simulink model "ned2lla_block"  (R2024b)
settings: Solver=VariableStepAuto  StartTime=0.0  StopTime=15  RelTol=1e-3
libraries: simulink x6, aerolibfltsims x1
settings Model: Creator=victo  LastModifiedBy=victo

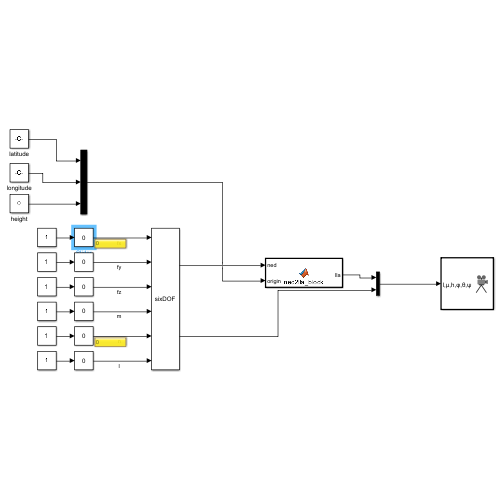
[thumbnail: Simulink's stored preview of the top-level diagram]
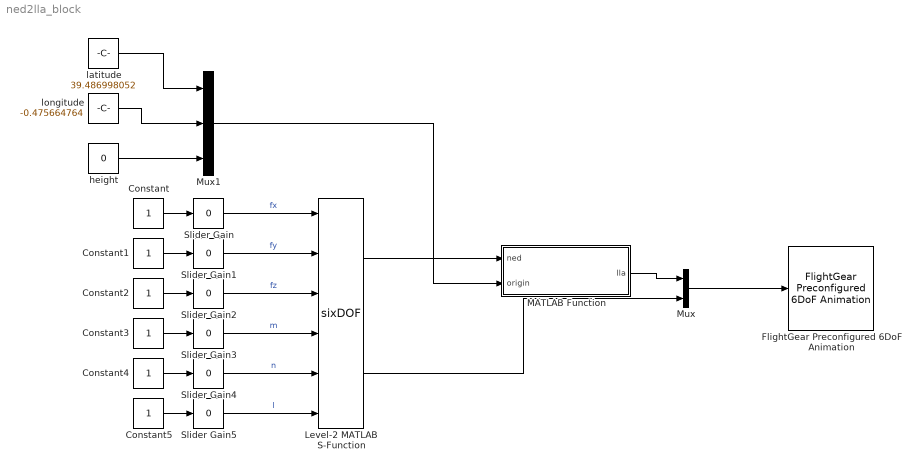
== system ned2lla_block ==
  Constant{,1..5} (6 alike) : Constant
  FlightGear Preconfigured 6DoF Animation : aerolibfltsims/FlightGear Preconfigured 6DoF Animation  xFlightGearVersion=v2019.1  DestinationIpAddress=127.0.0.1  DestinationPort=5501  SampleTime=1/30  packetVersion=24
  Level-2 MATLAB S-Function : M-S-Function  FunctionName=sixDOF
  MATLAB Function : MATLAB Function  TreatAsAtomicUnit=on
  Mux : Mux  Inputs=2
  Mux1 : Mux  Inputs=3
  Slider Gain{,1..5} (6 alike) : simulink/Math Operations/Slider Gain  gain=0  low=-5  high=5
  height : Constant  Value=0
  latitude : Constant  Value=39.486998052
  longitude : Constant  Value=-0.475664764
  wires:
  Slider Gain5/1 -> Level-2 MATLAB S-Function/6  "l"
  Slider Gain4/1 -> Level-2 MATLAB S-Function/5  "n"
  Slider Gain3/1 -> Level-2 MATLAB S-Function/4  "m"
  Slider Gain2/1 -> Level-2 MATLAB S-Function/3  "fz"
  Slider Gain1/1 -> Level-2 MATLAB S-Function/2  "fy"
  Slider Gain/1 -> Level-2 MATLAB S-Function/1  "fx"
  Constant/1 -> Slider Gain/1
  Constant1/1 -> Slider Gain1/1
  Constant2/1 -> Slider Gain2/1
  Constant3/1 -> Slider Gain3/1
  Constant4/1 -> Slider Gain4/1
  Constant5/1 -> Slider Gain5/1
  Level-2 MATLAB S-Function/1 -> MATLAB Function/1(ned)
  Level-2 MATLAB S-Function/2 -> Mux/2
  MATLAB Function/1(lla) -> Mux/1
  latitude/1 -> Mux1/1
  height/1 -> Mux1/3
  longitude/1 -> Mux1/2
  Mux1/1 -> MATLAB Function/2(origin)
  Mux/1 -> FlightGear Preconfigured 6DoF Animation/1

== matlab function ned2lla_block/MATLAB Function ==
  data: ned input; lla output; origin input
function lla = ned2lla_block(ned,origin)
lla=ned2lla(ned',origin',"ellipsoid");
aux=lla(1);
lla(1)=lla(2);
lla(2)=aux;
